simulink model "labview_control_loop"  (R2013a)
settings: Solver=ode45  StartTime=0.0  StopTime=10.0  RelTol=1e-3
libraries: simulink x1
settings Model: Creator=mainster  LastModifiedBy=mainster

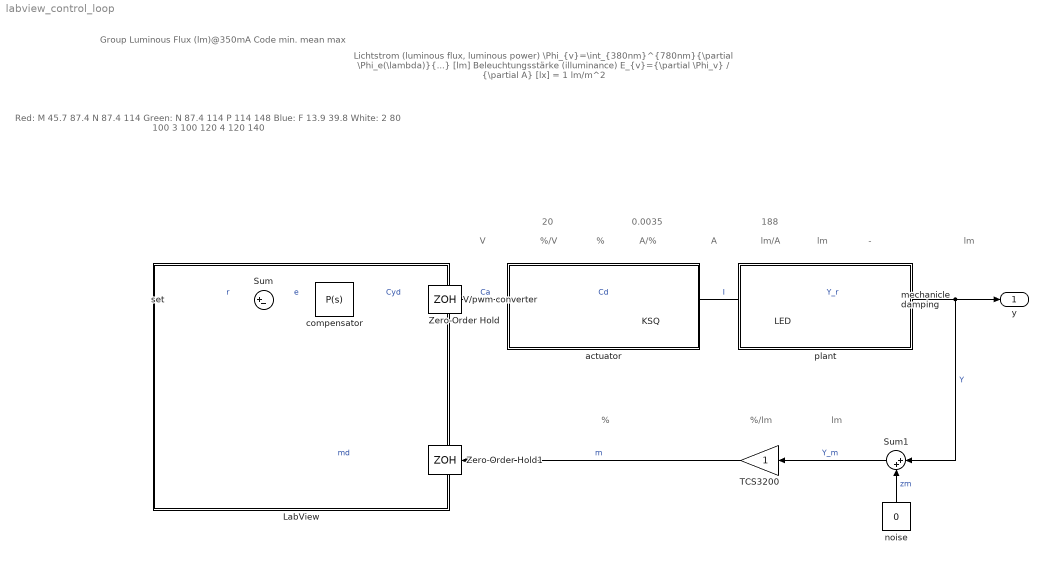
== system labview_control_loop ==
  note: Group	Luminous Flux (lm)@350mA
      |  Code  	min.		mean		max
  note: Red:		M		45.7		87.4
      | 			N 		87.4 		114
      | Green:	N 		87.4 		114
      | 			P 		114 		148
      | Blue:		F 		13.9 		39.8
      | White:		2 		80 			100
      | 			3 		100 		120
      | 			4 		120 		140
  note: Lichtstrom
      | (luminous flux,
      | luminous power)		\Phi_{v}=\int_{380nm}^{780nm}{\partial \Phi_e(\lambda)}{...}		 [lm]
      | Beleuchtungsstärke
      | (illuminance)				E_{v}={\partial \Phi_v} / {\partial A}		 		[lx] = 1 lm/m^2
  note: V
  note: %/V
  note: %
  note: A/%
  note: A
  note: lm/A
  note: lm
  note: -
  note: lm
  note: lm
  note: %
  note: %/lm
  note: 20
  note: 0.0035
  note: 188
  set : Inport
  KSQ : Gain  Gain=0.0035
  LED : Gain  Gain=188
  LabView : Subsystem
      mask Display: disp('')
  Sum : Sum  Inputs=|+-
  Sum1 : Sum  Inputs=|++
  TCS3200 : Gain
  V/pwm converter : Gain  Gain=20
  Zero-Order Hold : ZeroOrderHold
  Zero-Order Hold1 : ZeroOrderHold
  actuator : Subsystem
      mask Display: disp('')
  compensator : simulink/Continuous/PID Controller  Controller=P  TimeDomain=Continuous-time  SampleTime=1  IntegratorMethod=Forward Euler  FilterMethod=Forward Euler  Form=Parallel  P=1  I=1  D=0  N=100  InitialConditionSource=internal  InitialConditionForIntegrator=0  InitialConditionForFilter=0  ExternalReset=none  LimitOutput=off  UpperSaturationLimit=inf  LowerSaturationLimit=-inf  LinearizeAsGain=on  AntiWindupMode=none  Kb=1  TrackingMode=off  Kt=1  PParamMin=[]  PParamMax=[]  IParamMin=[]  IParamMax=[]  DParamMin=[]  DParamMax=[]  NParamMin=[]  NParamMax=[]  KbParamMin=[]  KbParamMax=[]  KtParamMin=[]  KtParamMax=[]  POutMin=[]  POutMax=[]  IOutMin=[]  IOutMax=[]  DOutMin=[]  DOutMax=[]  NOutMin=[]  NOutMax=[]  KbOutMin=[]  KbOutMax=[]  KtOutMin=[]  KtOutMax=[]  IntegratorOutMin=[]  IntegratorOutMax=[]  FilterOutMin=[]  FilterOutMax=[]  SumOutMin=[]  SumOutMax=[]  SumI1OutMin=[]  SumI1OutMax=[]  SumI2OutMin=[]  SumI2OutMax=[]  SumI3OutMin=[]  SumI3OutMax=[]  SumDOutMin=[]  SumDOutMax=[]  SaturationOutMin=[]  SaturationOutMax=[]  IntegratorContinuousStateAttributes=''  IntegratorStateMustResolveToSignalObject=off  IntegratorRTWStateStorageClass=Auto  FilterContinuousStateAttributes=''  FilterStateMustResolveToSignalObject=off  FilterRTWStateStorageClass=Auto  mask(PID 1dof){}
      mask Display:
      | % This is a new mask on top of the base mask.
      | % Use "View base mask" link below to see the base mask.
      | fprintf('C(s)\nP/PI')
  mechanicle damping : Gain
  noise : Constant  Value=0
  plant : Subsystem
      mask Display: disp('')
  y : Outport
  wires:
  Sum/1 -> compensator/1  "e"
  compensator/1 -> Zero-Order Hold/1  "Cyd"
  Zero-Order Hold/1 -> V/pwm converter/1  "Ca"
  V/pwm converter/1 -> KSQ/1  "Cd"
  KSQ/1 -> LED/1  "I"
  mechanicle damping/1 -> y/1, Sum1/1  "Y"
  noise/1 -> Sum1/2  "zm"
  Sum1/1 -> TCS3200/1  "Y_m"
  LED/1 -> mechanicle damping/1  "Y_r"
  TCS3200/1 -> Zero-Order Hold1/1  "m"
  set/1 -> Sum/1  "r"
  Zero-Order Hold1/1 -> Sum/2  "md"

== system labview_control_loop/LabView ==

== system labview_control_loop/actuator ==

== system labview_control_loop/plant ==
